simulink model "PSKfilter"  (R2019a)
settings: Solver=VariableStepDiscrete  StartTime=0.0  StopTime=0.1  RelTol=1e-3
undefined symbols (not defined in the file): gcbh, rcfiltgaincompat
libraries: commdigbbndpm3 x2, commfilt2 x2, commchan3 x1, commrandsrc3 x1, commsink2 x1, commrflib2 x1, simulink x1, dspmathops x1
settings Model: Creator=giannis  LastModifiedBy=giannis

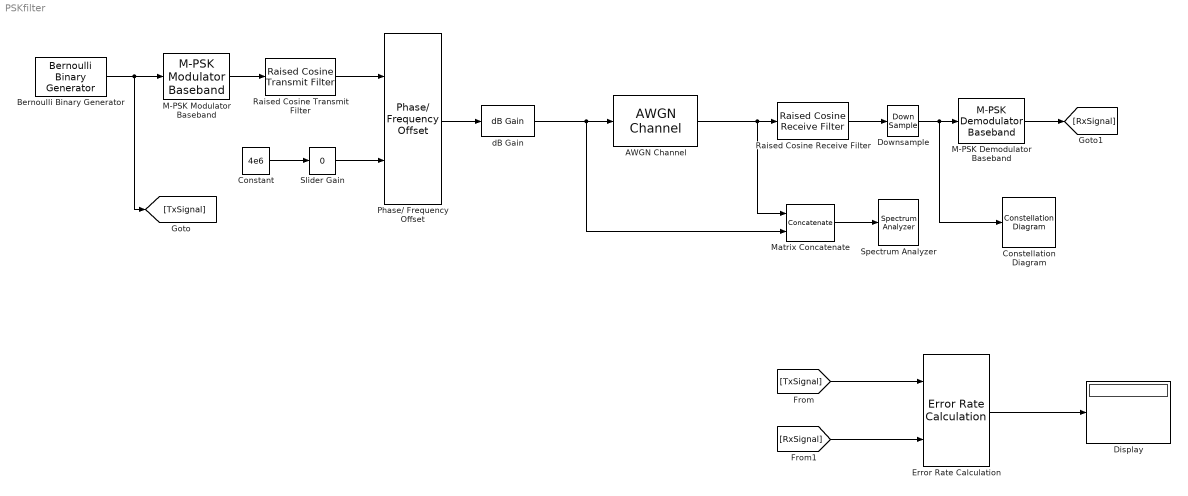
== system PSKfilter ==
  AWGN Channel : commchan3/AWGN Channel  InputProcessing=Columns as channels (frame based)  seed=123456  noiseMode="Signal to noise ratio  (SNR)"  EbNodB=10  EsNodB=10  SNRdB=8  bitsPerSym=1  Ps=1/8  Tsym=1  variance=1
      settings: SourceProductName=Communications Toolbox
  Bernoulli Binary Generator : commrandsrc3/Bernoulli Binary Generator  ProbabilityOfZero=0.5  SeedSource=Parameter  Seed=529558  SampleTime=1e-6/3  SamplesPerFrame=300  OutputDataType=boolean  SimulateUsing=Interpreted execution
      settings: SourceProductName=Communications Toolbox
  Constant : Constant  Value=4e6  SampleTime=(1e-6/3)*300
  Constellation Diagram : ConstellationDiagram
  Display : Display
  Downsample : DownSample  N=8
  Error Rate Calculation : commsink2/Error Rate Calculation  N=12*3  st_delay=0  cp_mode=Entire frame  subframe=[]  PMode=Port  WsName=ErrorVec  RsMode2=off  stop=off  numErr=100  maxBits=1e6
      settings: SourceProductName=Communications Toolbox
  M-PSK Demodulator Baseband : commdigbbndpm3/M-PSK Demodulator Baseband  M=8  OutType=Bit  DecType=Hard decision  VarSource=Dialog  Variance=1  Dec=Gray  Mapping=[0:7]  Ph=0  outDtype1=boolean  outDtype2=Inherit via internal rule  derotateFactorWordLen=16  derotateFactorDataTypeStr=Inherit: Same word length as input  derotateFactorLastDataTypeStr=Inherit: Same word length as input
      settings: SourceProductName=Communications Toolbox
  M-PSK Modulator Baseband : commdigbbndpm3/M-PSK Modulator Baseband  M=8  InType=Bit  Enc=Gray  Mapping=[0:7]  Ph=0  outDtype=double  outWordLen=16  outUDDataType=sfix(16)  outFracLenMode=Best precision  outFracLen=15  outDataTypeStr=double  outLastDataTypeStr=double
      settings: SourceProductName=Communications Toolbox
  Matrix Concatenate : Concatenate  Mode=Multidimensional array  ConcatenateDimension=2
  Phase/ Frequency Offset : commrflib2/Phase// Frequency Offset  phaseOffset=0  freqPort=on  freqOffset=0
      settings: SourceProductName=Communications Toolbox
  Raised Cosine Receive Filter : commfilt2/Raised Cosine Receive Filter  filtType=Square root  R=0  filtSpan=2*(6)  N=8  downFactor=1  downOffset=0  filterGain=rcfiltgaincompat(gcbh)  InputProcessing=Columns as channels (frame based)  RateOptions=Enforce single-rate processing  framing=Mute  checkCoeff=off  variableName=rcRxFilt  currentFiltSpan=2*(6)  D=(2*(6))/2  inputOffset=0  sampMode=Mute  saveAsFlag=0  rateMode=Downsampling  checkGain=Normalized  launchFVT=on  roundingMode=Floor  overflowMode=off  coeffDataTypeStr=Inherit: Same word length as input  coeffMin=[]  coeffMax=[]  coeffLastDataTypeStr=Inherit: Same word length as input  accumDataTypeStr=Inherit: Same as product output  accumLastDataTypeStr=Inherit: Same as product output  outputDataTypeStr=Inherit: Same as accumulator  outputMin=[]  outputMax=[]  outputLastDataTypeStr=Inherit: Same as accumulator
      settings: SourceProductName=Communications Toolbox
  Raised Cosine Transmit Filter : commfilt2/Raised Cosine Transmit Filter  filtType=Square root  R=0  filtSpan=2*(6)  N=8  filterGain=rcfiltgaincompat(gcbh)  InputProcessing=Columns as channels (frame based)  RateOptions=Enforce single-rate processing  framing=Mute  checkCoeff=off  variableName=rcTxFilt  checkGain=Normalized  sampMode=Mute  saveAsFlag=0  currentFiltSpan=2*(6)  D=(2*(6))/2  launchFVT=on  roundingMode=Floor  overflowMode=off  coeffDataTypeStr=Inherit: Same word length as input  coeffMin=[]  coeffMax=[]  coeffLastDataTypeStr=Inherit: Same word length as input  outputDataTypeStr=Inherit: Same as accumulator  outputMin=[]  outputMax=[]  outputLastDataTypeStr=Inherit: Same as accumulator
      settings: SourceProductName=Communications Toolbox
  Slider Gain : simulink/Math Operations/Slider Gain  gain=0  low=-2  high=2
  Spectrum Analyzer : SpectrumAnalyzer
  dB Gain : dspmathops/dB Gain  dB=0  intype=Amplitude
      settings: SourceProductName=DSP System Toolbox  SourceProductBaseCode=DS
  wires:
  Bernoulli Binary Generator/1 -> [TxSignal], M-PSK Modulator Baseband/1
  M-PSK Modulator Baseband/1 -> Raised Cosine Transmit Filter/1
  Raised Cosine Transmit Filter/1 -> Phase/ Frequency Offset/1
  Constant/1 -> Slider Gain/1
  Phase/ Frequency Offset/1 -> dB Gain/1
  Slider Gain/1 -> Phase/ Frequency Offset/2
  dB Gain/1 -> Matrix Concatenate/2, AWGN Channel/1
  AWGN Channel/1 -> Matrix Concatenate/1, Raised Cosine Receive Filter/1
  Raised Cosine Receive Filter/1 -> Downsample/1
  Downsample/1 -> Constellation Diagram/1, M-PSK Demodulator Baseband/1
  M-PSK Demodulator Baseband/1 -> [RxSignal]
  Matrix Concatenate/1 -> Spectrum Analyzer/1
  Error Rate Calculation/1 -> Display/1
  [TxSignal] -> Error Rate Calculation/1
  [RxSignal] -> Error Rate Calculation/2
